simulink model "try_place"  (R2018b)
settings: Solver=VariableStepAuto  StartTime=0.0  StopTime=15  RelTol=1e-3
values from neighbouring files (symbols this model uses):
  A = [0,1;0,0]    [AAAA_trying.m]    (also in MPCController.m = plant.A; MPCController1.m; aaass.m; app1.m = 1)
  b = [0;1]    [AAAA_trying.m]    (also in aaass.m)
  cT = [1,0]    [aaass.m]
undefined symbols (not defined in the file or in its folder): K
settings Model: Creator=HP  LastModifiedBy=HP

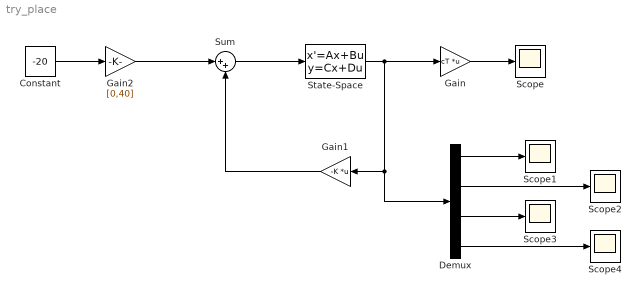
== system try_place ==
  Constant : Constant  Value=-20
  Demux : Demux
  Gain : Gain  Gain=cT  Multiplication=Matrix(K*u)
  Gain1 : Gain  Gain=-K  Multiplication=Matrix(K*u)
  Gain2 : Gain  Gain=[0,40]
  Scope{,1..4} (5 alike) : Scope
  State-Space : StateSpace  A=A  B=b  C=eye(4)  D=zeros(4,2)  InitialCondition=[0;-80;20;25]
  Sum : Sum  Inputs=|++
  wires:
  State-Space/1 -> Gain/1, Demux/1, Gain1/1
  Sum/1 -> State-Space/1
  Gain1/1 -> Sum/2
  Gain2/1 -> Sum/1
  Constant/1 -> Gain2/1
  Gain/1 -> Scope/1
  Demux/1 -> Scope1/1
  Demux/2 -> Scope2/1
  Demux/3 -> Scope3/1
  Demux/4 -> Scope4/1
